simulink library "LibDBC_VCUa_ch1"  (R2024b)
settings: Solver=VariableStepAuto  StartTime=0.0  StopTime=10.0  RelTol=1e-3
undefined symbols (not defined in the file): bit_packing, IO_Blk_Lib_TTC500, IO_CAN_ConfigMsg
libraries: IOBlock_Library_TTC580 x2, simulink x2
(part 1 of 2)
Description:
  | 13-Jun-2024 19:00:134624
settings Model: Creator=Jacob  LastModifiedBy=Jacob

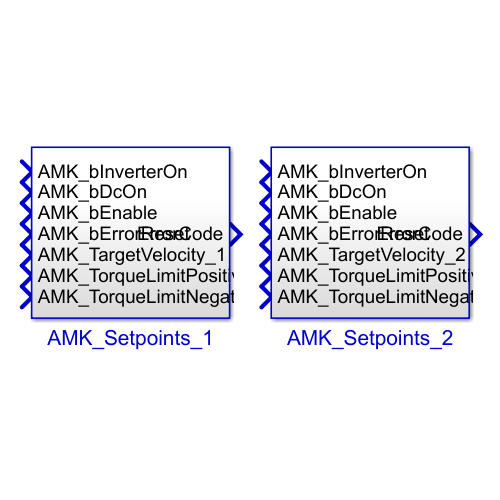
[thumbnail: Simulink's stored preview of the top-level diagram]
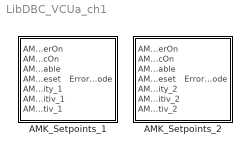
== system LibDBC_VCUa_ch1 ==
  AMK_Setpoints_1 : Subsystem  Priority=0
  AMK_Setpoints_2 : Subsystem  Priority=0

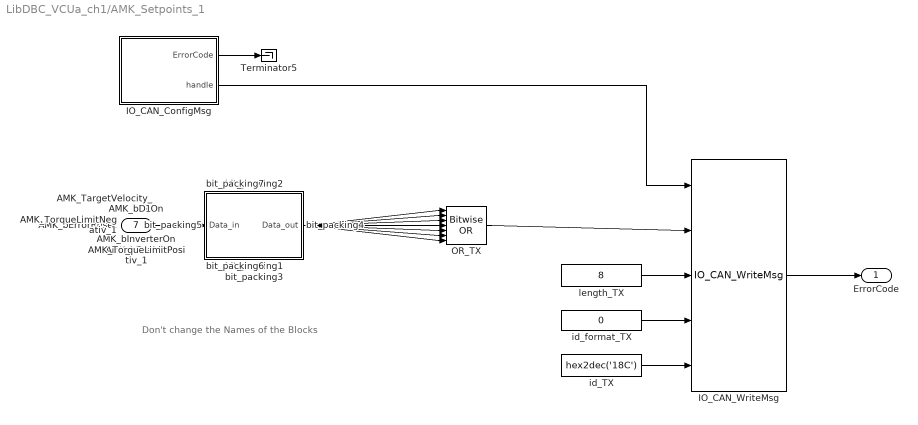
== system LibDBC_VCUa_ch1/AMK_Setpoints_1 ==
  note: Don't change the Names of the Blocks
  AMK_bInverterOn : Inport
  AMK_bDcOn : Inport  Port=2
  AMK_bEnable : Inport  Port=3
  AMK_bErrorReset : Inport  Port=4
  AMK_TargetVelocity_1 : Inport  Port=5
  AMK_TorqueLimitPositiv_1 : Inport  Port=6
  AMK_TorqueLimitNegativ_1 : Inport  Port=7
  IO_CAN_ConfigMsg : Subsystem  mask(IO_CAN_ConfigMsg_Code){SampleTime=-1, ttlib=IO_Blk_Lib_TTC500, ttDescription=IO_CAN_ConfigMsg, tt_iolib_version=0.19, channel=IO_CAN_CHANNEL_1, mode=IO_CAN_MSG_WRITE, id_format=IO_CAN_STD_FRAME, id=0x18C, ac_mask=0x7FF}
      mask help: Configures a message object for the given CAN channel.
      mask init:
      | %
      mask Help: web(which('IO_CAN.h'))
      mask TypeOptions channel: IO_CAN_CHANNEL_0  | IO_CAN_CHANNEL_1 | IO_CAN_CHANNEL_2 | IO_CAN_CHANNEL_3 | IO_CAN_CHANNEL_4 | IO_CAN_CHANNEL_5 | IO_CAN_CHANNEL_6
      mask Callback channel: %
      mask TypeOptions mode: IO_CAN_MSG_READ | IO_CAN_MSG_WRITE
      mask Callback mode: %
      mask TypeOptions id_format: IO_CAN_STD_FRAME | IO_CAN_EXT_FRAME
      mask Callback id_format: %
      mask Callback id: %
      mask Callback ac_mask: %
  IO_CAN_WriteMsg : IOBlock_Library_TTC580/CAN  Blocks TTC580 IOlib/WriteMsg_CAN/IO_CAN_WriteMsg  SampleTime=-1  ttlib=IO_Blk_Lib_TTC500  ttDescription=IO_CAN_WriteMsg  tt_iolib_version=0.19
      settings: SourceProductName=I/O Blocklibrary for TTC580
  OR_TX : simulink/Logic and Bit Operations/Bitwise Operator  logicop=OR  UseBitMask=off  NumInputPorts=7  BitMask=bin2dec('11011001')  BitMaskRealWorld=Stored Integer
  Terminator5 : Terminator
  bit_packing1 : Subsystem  LoadFcn=|  mask(bit_packing_Code){SampleTime=-1, ttlib=IO_Blk_Lib_TTC500, ttDescription=bit_packing, tt_iolib_version=0.26, Endianness=little, Format=unsigned, Inversion=off, Startbit=8, Width_bits=1, Factor=1, Offset=0}
      | try
      | %
      | %Upgrade Information - standard BEGIN
      | new_color = 'blue';
      | new_ver = '0.26';
      | act_ver = get_param(gcb,'tt_iolib_version');
      | if not(strcmp(act_ver,new_ver))
      |     disp(['Upgrade block: ',gcb,char(10),'       Version: ',act_ver,' to ',new_ver]);
      |     %switch - case for specific upgrade information e.g. additional parameter required 
      |     %Change appearance and version information
      |     set_param(gcb,'ForegroundColor',new_color);
      |     set_param(gcb,'tt_iolib_version',new_ver);
      | end
      | %Upgrade Information - standard END
      | catch
      | %Standard catch section BEGIN
      | errordlg('An error occurred in a callback of the TTC580-BlockLib. Please open the Diagnostic Viewer for further details');
      | disp(' ');
      | disp('------------------------------------------------------------');
      | disp('An error occurred in a callback of the TTC580-BlockLib.');
      | disp(['Please check the parameters in the mask of ',gcb]);
      | disp('If you do not encounter any violations, then please '); 
      | disp('copy the following lines and report this to support@ttcontrol.com ');
      | disp('<< begin of error message dump >>');
      | disp(['Version of TTC580-BlockLib: ', get_param(gcb,'tt_iolib_version')]);
      | disp(get_param(gcb,'ttDescription'));
      | disp(gcb);
      | x=lasterror;disp(x.message);
      | disp(get_param(gcb,'MaskValues'));
      | disp(version);
      | disp(computer);
      | disp('<< end of error message dump >>');
      | disp('------------------------------------------------------------');
      | disp(' ');
      | %Standard catch section END
      | end
      mask help:
      | Block to prepare CAN-transmition at specified position within 64bit field.
      | For "Factor" and "Offset" the definition of Vector's CANdb applies:
      | [Physical value] = ( [Raw value] * [Factor] ) + [Offset]
      | with Raw value of a signal being the value as it is transmitted in the CAN-network.
      | Verification capabilities are supported.
      mask init:
      | try
      | %%CT>
      | TAG_loc = get_param(gcb,'Tag');
      | if ~isempty(TAG_loc),[~,y]=regexp(TAG_loc,'(^[a-zA-Z0-9_]*)');
      |     if isempty(y) || y~=builtin('length',(TAG_loc)) %don't use length() alone!
      |         error(['The Tag: ',TAG_loc,' needs to start with a letter and may only contain the characters 0-9,a-Z,_ .']);
      | end,end
      | x=find_system(gcbh,'FollowLinks','on','LookUnderMasks','on','BlockType','S-Function');
      | for i=1:builtin('length',(x)) %don't use length() alone!
      |     set_param(x(i),'Tag',TAG_loc);
      | end
      | %<CT%
      | 
      | catch
      | %Standard catch section BEGIN
      | errordlg('An error occurred in a callback of the TTC580-BlockLib. Please open the Diagnostic Viewer for further details');
      | disp(' ');
      | disp('------------------------------------------------------------');
      | disp('An error occurred in a callback of the TTC580-BlockLib.');
      | disp(['Please check the parameters in the mask of ',gcb]);
      | disp('If you do not encounter any violations, then please '); 
      | disp('copy the following lines and report this to support@ttcontrol.com ');
      | disp('<< begin of error message dump >>');
      | disp(['Version of TTC580-BlockLib: ', get_param(gcb,'tt_iolib_version')]);
      | disp(get_param(gcb,'ttDescription'));
      | disp(gcb);
      | x=lasterror;disp(x.message);
      | disp(get_param(gcb,'MaskValues'));
      | disp(version);
      | disp(computer);
      | disp('<< end of error message dump >>');
      | disp('------------------------------------------------------------');
      | disp(' ');
      | %Standard catch section END
      | end
      mask Help: web([which('usermanual.html'),'#',lower(get_param(gcb,'ttDescription'))])
      mask TypeOptions Endianness: big | little
      mask Callback Endianness: %
      mask TypeOptions Format: unsigned | signed | real32
      mask Callback Format: %
      mask Callback Inversion: %
      mask Callback Startbit: %
      mask Callback Width_bits: %
      mask Callback Factor: %
      mask Callback Offset: %
  bit_packing2 : Subsystem  LoadFcn=|  mask(bit_packing_Code){SampleTime=-1, ttlib=IO_Blk_Lib_TTC500, ttDescription=bit_packing, tt_iolib_version=0.26, Endianness=little, Format=unsigned, Inversion=off, Startbit=9, Width_bits=1, Factor=1, Offset=0}
      | try
      | %
      | %Upgrade Information - standard BEGIN
      | new_color = 'blue';
      | new_ver = '0.26';
      | act_ver = get_param(gcb,'tt_iolib_version');
      | if not(strcmp(act_ver,new_ver))
      |     disp(['Upgrade block: ',gcb,char(10),'       Version: ',act_ver,' to ',new_ver]);
      |     %switch - case for specific upgrade information e.g. additional parameter required 
      |     %Change appearance and version information
      |     set_param(gcb,'ForegroundColor',new_color);
      |     set_param(gcb,'tt_iolib_version',new_ver);
      | end
      | %Upgrade Information - standard END
      | catch
      | %Standard catch section BEGIN
      | errordlg('An error occurred in a callback of the TTC580-BlockLib. Please open the Diagnostic Viewer for further details');
      | disp(' ');
      | disp('------------------------------------------------------------');
      | disp('An error occurred in a callback of the TTC580-BlockLib.');
      | disp(['Please check the parameters in the mask of ',gcb]);
      | disp('If you do not encounter any violations, then please '); 
      | disp('copy the following lines and report this to support@ttcontrol.com ');
      | disp('<< begin of error message dump >>');
      | disp(['Version of TTC580-BlockLib: ', get_param(gcb,'tt_iolib_version')]);
      | disp(get_param(gcb,'ttDescription'));
      | disp(gcb);
      | x=lasterror;disp(x.message);
      | disp(get_param(gcb,'MaskValues'));
      | disp(version);
      | disp(computer);
      | disp('<< end of error message dump >>');
      | disp('------------------------------------------------------------');
      | disp(' ');
      | %Standard catch section END
      | end
      mask help:
      | Block to prepare CAN-transmition at specified position within 64bit field.
      | For "Factor" and "Offset" the definition of Vector's CANdb applies:
      | [Physical value] = ( [Raw value] * [Factor] ) + [Offset]
      | with Raw value of a signal being the value as it is transmitted in the CAN-network.
      | Verification capabilities are supported.
      mask init: same as LibDBC_VCUa_ch1/AMK_Setpoints_1/bit_packing1
      mask Help: web([which('usermanual.html'),'#',lower(get_param(gcb,'ttDescription'))])
      mask TypeOptions Endianness: big | little
      mask Callback Endianness: %
      mask TypeOptions Format: unsigned | signed | real32
      mask Callback Format: %
      mask Callback Inversion: %
      mask Callback Startbit: %
      mask Callback Width_bits: %
      mask Callback Factor: %
      mask Callback Offset: %
  bit_packing3 : Subsystem  LoadFcn=|  mask(bit_packing_Code){SampleTime=-1, ttlib=IO_Blk_Lib_TTC500, ttDescription=bit_packing, tt_iolib_version=0.26, Endianness=little, Format=unsigned, Inversion=off, Startbit=10, Width_bits=1, Factor=1, Offset=0}
      | try
      | %
      | %Upgrade Information - standard BEGIN
      | new_color = 'blue';
      | new_ver = '0.26';
      | act_ver = get_param(gcb,'tt_iolib_version');
      | if not(strcmp(act_ver,new_ver))
      |     disp(['Upgrade block: ',gcb,char(10),'       Version: ',act_ver,' to ',new_ver]);
      |     %switch - case for specific upgrade information e.g. additional parameter required 
      |     %Change appearance and version information
      |     set_param(gcb,'ForegroundColor',new_color);
      |     set_param(gcb,'tt_iolib_version',new_ver);
      | end
      | %Upgrade Information - standard END
      | catch
      | %Standard catch section BEGIN
      | errordlg('An error occurred in a callback of the TTC580-BlockLib. Please open the Diagnostic Viewer for further details');
      | disp(' ');
      | disp('------------------------------------------------------------');
      | disp('An error occurred in a callback of the TTC580-BlockLib.');
      | disp(['Please check the parameters in the mask of ',gcb]);
      | disp('If you do not encounter any violations, then please '); 
      | disp('copy the following lines and report this to support@ttcontrol.com ');
      | disp('<< begin of error message dump >>');
      | disp(['Version of TTC580-BlockLib: ', get_param(gcb,'tt_iolib_version')]);
      | disp(get_param(gcb,'ttDescription'));
      | disp(gcb);
      | x=lasterror;disp(x.message);
      | disp(get_param(gcb,'MaskValues'));
      | disp(version);
      | disp(computer);
      | disp('<< end of error message dump >>');
      | disp('------------------------------------------------------------');
      | disp(' ');
      | %Standard catch section END
      | end
      mask help:
      | Block to prepare CAN-transmition at specified position within 64bit field.
      | For "Factor" and "Offset" the definition of Vector's CANdb applies:
      | [Physical value] = ( [Raw value] * [Factor] ) + [Offset]
      | with Raw value of a signal being the value as it is transmitted in the CAN-network.
      | Verification capabilities are supported.
      mask init: same as LibDBC_VCUa_ch1/AMK_Setpoints_1/bit_packing1
      mask Help: web([which('usermanual.html'),'#',lower(get_param(gcb,'ttDescription'))])
      mask TypeOptions Endianness: big | little
      mask Callback Endianness: %
      mask TypeOptions Format: unsigned | signed | real32
      mask Callback Format: %
      mask Callback Inversion: %
      mask Callback Startbit: %
      mask Callback Width_bits: %
      mask Callback Factor: %
      mask Callback Offset: %
  bit_packing4 : Subsystem  LoadFcn=|  mask(bit_packing_Code){SampleTime=-1, ttlib=IO_Blk_Lib_TTC500, ttDescription=bit_packing, tt_iolib_version=0.26, Endianness=little, Format=unsigned, Inversion=off, Startbit=11, Width_bits=1, Factor=1, Offset=0}
      | try
      | %
      | %Upgrade Information - standard BEGIN
      | new_color = 'blue';
      | new_ver = '0.26';
      | act_ver = get_param(gcb,'tt_iolib_version');
      | if not(strcmp(act_ver,new_ver))
      |     disp(['Upgrade block: ',gcb,char(10),'       Version: ',act_ver,' to ',new_ver]);
      |     %switch - case for specific upgrade information e.g. additional parameter required 
      |     %Change appearance and version information
      |     set_param(gcb,'ForegroundColor',new_color);
      |     set_param(gcb,'tt_iolib_version',new_ver);
      | end
      | %Upgrade Information - standard END
      | catch
      | %Standard catch section BEGIN
      | errordlg('An error occurred in a callback of the TTC580-BlockLib. Please open the Diagnostic Viewer for further details');
      | disp(' ');
      | disp('------------------------------------------------------------');
      | disp('An error occurred in a callback of the TTC580-BlockLib.');
      | disp(['Please check the parameters in the mask of ',gcb]);
      | disp('If you do not encounter any violations, then please '); 
      | disp('copy the following lines and report this to support@ttcontrol.com ');
      | disp('<< begin of error message dump >>');
      | disp(['Version of TTC580-BlockLib: ', get_param(gcb,'tt_iolib_version')]);
      | disp(get_param(gcb,'ttDescription'));
      | disp(gcb);
      | x=lasterror;disp(x.message);
      | disp(get_param(gcb,'MaskValues'));
      | disp(version);
      | disp(computer);
      | disp('<< end of error message dump >>');
      | disp('------------------------------------------------------------');
      | disp(' ');
      | %Standard catch section END
      | end
      mask help:
      | Block to prepare CAN-transmition at specified position within 64bit field.
      | For "Factor" and "Offset" the definition of Vector's CANdb applies:
      | [Physical value] = ( [Raw value] * [Factor] ) + [Offset]
      | with Raw value of a signal being the value as it is transmitted in the CAN-network.
      | Verification capabilities are supported.
      mask init: same as LibDBC_VCUa_ch1/AMK_Setpoints_1/bit_packing1
      mask Help: web([which('usermanual.html'),'#',lower(get_param(gcb,'ttDescription'))])
      mask TypeOptions Endianness: big | little
      mask Callback Endianness: %
      mask TypeOptions Format: unsigned | signed | real32
      mask Callback Format: %
      mask Callback Inversion: %
      mask Callback Startbit: %
      mask Callback Width_bits: %
      mask Callback Factor: %
      mask Callback Offset: %
  bit_packing5 : Subsystem  LoadFcn=|  mask(bit_packing_Code){SampleTime=-1, ttlib=IO_Blk_Lib_TTC500, ttDescription=bit_packing, tt_iolib_version=0.26, Endianness=little, Format=signed, Inversion=off, Startbit=16, Width_bits=16, Factor=1, Offset=0}
      | try
      | %
      | %Upgrade Information - standard BEGIN
      | new_color = 'blue';
      | new_ver = '0.26';
      | act_ver = get_param(gcb,'tt_iolib_version');
      | if not(strcmp(act_ver,new_ver))
      |     disp(['Upgrade block: ',gcb,char(10),'       Version: ',act_ver,' to ',new_ver]);
      |     %switch - case for specific upgrade information e.g. additional parameter required 
      |     %Change appearance and version information
      |     set_param(gcb,'ForegroundColor',new_color);
      |     set_param(gcb,'tt_iolib_version',new_ver);
      | end
      | %Upgrade Information - standard END
      | catch
      | %Standard catch section BEGIN
      | errordlg('An error occurred in a callback of the TTC580-BlockLib. Please open the Diagnostic Viewer for further details');
      | disp(' ');
      | disp('------------------------------------------------------------');
      | disp('An error occurred in a callback of the TTC580-BlockLib.');
      | disp(['Please check the parameters in the mask of ',gcb]);
      | disp('If you do not encounter any violations, then please '); 
      | disp('copy the following lines and report this to support@ttcontrol.com ');
      | disp('<< begin of error message dump >>');
      | disp(['Version of TTC580-BlockLib: ', get_param(gcb,'tt_iolib_version')]);
      | disp(get_param(gcb,'ttDescription'));
      | disp(gcb);
      | x=lasterror;disp(x.message);
      | disp(get_param(gcb,'MaskValues'));
      | disp(version);
      | disp(computer);
      | disp('<< end of error message dump >>');
      | disp('------------------------------------------------------------');
      | disp(' ');
      | %Standard catch section END
      | end
      mask help:
      | Block to prepare CAN-transmition at specified position within 64bit field.
      | For "Factor" and "Offset" the definition of Vector's CANdb applies:
      | [Physical value] = ( [Raw value] * [Factor] ) + [Offset]
      | with Raw value of a signal being the value as it is transmitted in the CAN-network.
      | Verification capabilities are supported.
      mask init: same as LibDBC_VCUa_ch1/AMK_Setpoints_1/bit_packing1
      mask Help: web([which('usermanual.html'),'#',lower(get_param(gcb,'ttDescription'))])
      mask TypeOptions Endianness: big | little
      mask Callback Endianness: %
      mask TypeOptions Format: unsigned | signed | real32
      mask Callback Format: %
      mask Callback Inversion: %
      mask Callback Startbit: %
      mask Callback Width_bits: %
      mask Callback Factor: %
      mask Callback Offset: %
  bit_packing6 : Subsystem  LoadFcn=|  mask(bit_packing_Code){SampleTime=-1, ttlib=IO_Blk_Lib_TTC500, ttDescription=bit_packing, tt_iolib_version=0.26, Endianness=little, Format=signed, Inversion=off, Startbit=32, Width_bits=16, Factor=1, Offset=0}
      | try
      | %
      | %Upgrade Information - standard BEGIN
      | new_color = 'blue';
      | new_ver = '0.26';
      | act_ver = get_param(gcb,'tt_iolib_version');
      | if not(strcmp(act_ver,new_ver))
      |     disp(['Upgrade block: ',gcb,char(10),'       Version: ',act_ver,' to ',new_ver]);
      |     %switch - case for specific upgrade information e.g. additional parameter required 
      |     %Change appearance and version information
      |     set_param(gcb,'ForegroundColor',new_color);
      |     set_param(gcb,'tt_iolib_version',new_ver);
      | end
      | %Upgrade Information - standard END
      | catch
      | %Standard catch section BEGIN
      | errordlg('An error occurred in a callback of the TTC580-BlockLib. Please open the Diagnostic Viewer for further details');
      | disp(' ');
      | disp('------------------------------------------------------------');
      | disp('An error occurred in a callback of the TTC580-BlockLib.');
      | disp(['Please check the parameters in the mask of ',gcb]);
      | disp('If you do not encounter any violations, then please '); 
      | disp('copy the following lines and report this to support@ttcontrol.com ');
      | disp('<< begin of error message dump >>');
      | disp(['Version of TTC580-BlockLib: ', get_param(gcb,'tt_iolib_version')]);
      | disp(get_param(gcb,'ttDescription'));
      | disp(gcb);
      | x=lasterror;disp(x.message);
      | disp(get_param(gcb,'MaskValues'));
      | disp(version);
      | disp(computer);
      | disp('<< end of error message dump >>');
      | disp('------------------------------------------------------------');
      | disp(' ');
      | %Standard catch section END
      | end
      mask help:
      | Block to prepare CAN-transmition at specified position within 64bit field.
      | For "Factor" and "Offset" the definition of Vector's CANdb applies:
      | [Physical value] = ( [Raw value] * [Factor] ) + [Offset]
      | with Raw value of a signal being the value as it is transmitted in the CAN-network.
      | Verification capabilities are supported.
      mask init: same as LibDBC_VCUa_ch1/AMK_Setpoints_1/bit_packing1
      mask Help: web([which('usermanual.html'),'#',lower(get_param(gcb,'ttDescription'))])
      mask TypeOptions Endianness: big | little
      mask Callback Endianness: %
      mask TypeOptions Format: unsigned | signed | real32
      mask Callback Format: %
      mask Callback Inversion: %
      mask Callback Startbit: %
      mask Callback Width_bits: %
      mask Callback Factor: %
      mask Callback Offset: %
  bit_packing7 : Subsystem  LoadFcn=|  mask(bit_packing_Code){SampleTime=-1, ttlib=IO_Blk_Lib_TTC500, ttDescription=bit_packing, tt_iolib_version=0.26, Endianness=little, Format=signed, Inversion=off, Startbit=48, Width_bits=16, Factor=0.01, Offset=0}
      | try
      | %
      | %Upgrade Information - standard BEGIN
      | new_color = 'blue';
      | new_ver = '0.26';
      | act_ver = get_param(gcb,'tt_iolib_version');
      | if not(strcmp(act_ver,new_ver))
      |     disp(['Upgrade block: ',gcb,char(10),'       Version: ',act_ver,' to ',new_ver]);
      |     %switch - case for specific upgrade information e.g. additional parameter required 
      |     %Change appearance and version information
      |     set_param(gcb,'ForegroundColor',new_color);
      |     set_param(gcb,'tt_iolib_version',new_ver);
      | end
      | %Upgrade Information - standard END
      | catch
      | %Standard catch section BEGIN
      | errordlg('An error occurred in a callback of the TTC580-BlockLib. Please open the Diagnostic Viewer for further details');
      | disp(' ');
      | disp('------------------------------------------------------------');
      | disp('An error occurred in a callback of the TTC580-BlockLib.');
      | disp(['Please check the parameters in the mask of ',gcb]);
      | disp('If you do not encounter any violations, then please '); 
      | disp('copy the following lines and report this to support@ttcontrol.com ');
      | disp('<< begin of error message dump >>');
      | disp(['Version of TTC580-BlockLib: ', get_param(gcb,'tt_iolib_version')]);
      | disp(get_param(gcb,'ttDescription'));
      | disp(gcb);
      | x=lasterror;disp(x.message);
      | disp(get_param(gcb,'MaskValues'));
      | disp(version);
      | disp(computer);
      | disp('<< end of error message dump >>');
      | disp('------------------------------------------------------------');
      | disp(' ');
      | %Standard catch section END
      | end
      mask help:
      | Block to prepare CAN-transmition at specified position within 64bit field.
      | For "Factor" and "Offset" the definition of Vector's CANdb applies:
      | [Physical value] = ( [Raw value] * [Factor] ) + [Offset]
      | with Raw value of a signal being the value as it is transmitted in the CAN-network.
      | Verification capabilities are supported.
      mask init: same as LibDBC_VCUa_ch1/AMK_Setpoints_1/bit_packing1
      mask Help: web([which('usermanual.html'),'#',lower(get_param(gcb,'ttDescription'))])
      mask TypeOptions Endianness: big | little
      mask Callback Endianness: %
      mask TypeOptions Format: unsigned | signed | real32
      mask Callback Format: %
      mask Callback Inversion: %
      mask Callback Startbit: %
      mask Callback Width_bits: %
      mask Callback Factor: %
      mask Callback Offset: %
  id_TX : Constant  Value=hex2dec('18C')  OutDataTypeStr=uint32
  id_format_TX : Constant  Value=0  OutDataTypeStr=Inherit: Inherit via back propagation
  length_TX : Constant  Value=8  OutDataTypeStr=Inherit: Inherit via back propagation
  ErrorCode : Outport  VectorParamsAs1DForOutWhenUnconnected=off
  wires:
  id_TX/1 -> IO_CAN_WriteMsg/5
  id_format_TX/1 -> IO_CAN_WriteMsg/4
  length_TX/1 -> IO_CAN_WriteMsg/3
  IO_CAN_ConfigMsg/2(handle) -> IO_CAN_WriteMsg/1
  IO_CAN_ConfigMsg/1(ErrorCode) -> Terminator5/1
  IO_CAN_WriteMsg/1 -> ErrorCode/1
  AMK_bInverterOn/1 -> bit_packing1/1(Data_in)
  bit_packing1/1(Data_out) -> OR_TX/1
  AMK_bDcOn/1 -> bit_packing2/1(Data_in)
  bit_packing2/1(Data_out) -> OR_TX/2
  AMK_bEnable/1 -> bit_packing3/1(Data_in)
  bit_packing3/1(Data_out) -> OR_TX/3
  AMK_bErrorReset/1 -> bit_packing4/1(Data_in)
  bit_packing4/1(Data_out) -> OR_TX/4
  AMK_TargetVelocity_1/1 -> bit_packing5/1(Data_in)
  bit_packing5/1(Data_out) -> OR_TX/5
  AMK_TorqueLimitPositiv_1/1 -> bit_packing6/1(Data_in)
  bit_packing6/1(Data_out) -> OR_TX/6
  AMK_TorqueLimitNegativ_1/1 -> bit_packing7/1(Data_in)
  bit_packing7/1(Data_out) -> OR_TX/7
  OR_TX/1 -> IO_CAN_WriteMsg/2

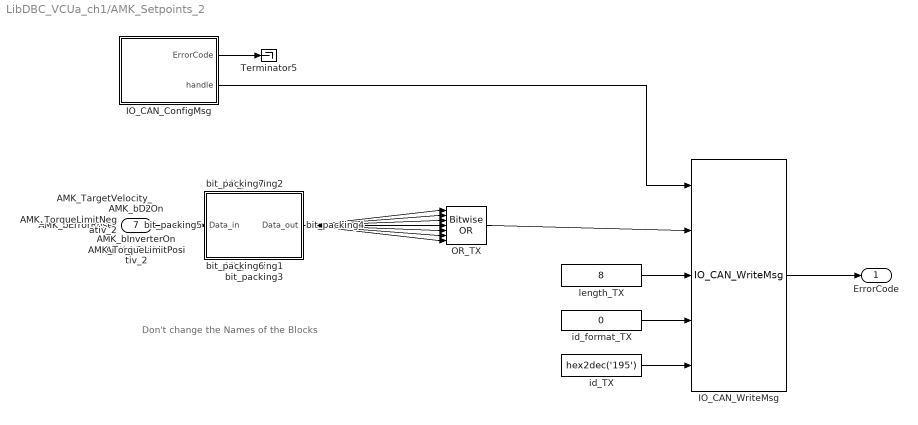
== system LibDBC_VCUa_ch1/AMK_Setpoints_2 ==
  note: Don't change the Names of the Blocks
  AMK_bInverterOn : Inport
  AMK_bDcOn : Inport  Port=2
  AMK_bEnable : Inport  Port=3
  AMK_bErrorReset : Inport  Port=4
  AMK_TargetVelocity_2 : Inport  Port=5
  AMK_TorqueLimitPositiv_2 : Inport  Port=6
  AMK_TorqueLimitNegativ_2 : Inport  Port=7
  IO_CAN_ConfigMsg : Subsystem  mask(IO_CAN_ConfigMsg_Code){SampleTime=-1, ttlib=IO_Blk_Lib_TTC500, ttDescription=IO_CAN_ConfigMsg, tt_iolib_version=0.19, channel=IO_CAN_CHANNEL_1, mode=IO_CAN_MSG_WRITE, id_format=IO_CAN_STD_FRAME, id=0x195, ac_mask=0x7FF}
      mask help: Configures a message object for the given CAN channel.
      mask init:
      | %
      mask Help: web(which('IO_CAN.h'))
      mask TypeOptions channel: IO_CAN_CHANNEL_0  | IO_CAN_CHANNEL_1 | IO_CAN_CHANNEL_2 | IO_CAN_CHANNEL_3 | IO_CAN_CHANNEL_4 | IO_CAN_CHANNEL_5 | IO_CAN_CHANNEL_6
      mask Callback channel: %
      mask TypeOptions mode: IO_CAN_MSG_READ | IO_CAN_MSG_WRITE
      mask Callback mode: %
      mask TypeOptions id_format: IO_CAN_STD_FRAME | IO_CAN_EXT_FRAME
      mask Callback id_format: %
      mask Callback id: %
      mask Callback ac_mask: %
  IO_CAN_WriteMsg : IOBlock_Library_TTC580/CAN  Blocks TTC580 IOlib/WriteMsg_CAN/IO_CAN_WriteMsg  SampleTime=-1  ttlib=IO_Blk_Lib_TTC500  ttDescription=IO_CAN_WriteMsg  tt_iolib_version=0.19
      settings: SourceProductName=I/O Blocklibrary for TTC580
  OR_TX : simulink/Logic and Bit Operations/Bitwise Operator  logicop=OR  UseBitMask=off  NumInputPorts=7  BitMask=bin2dec('11011001')  BitMaskRealWorld=Stored Integer
  Terminator5 : Terminator
  bit_packing1 : Subsystem  LoadFcn=|  mask(bit_packing_Code){SampleTime=-1, ttlib=IO_Blk_Lib_TTC500, ttDescription=bit_packing, tt_iolib_version=0.26, Endianness=little, Format=unsigned, Inversion=off, Startbit=8, Width_bits=1, Factor=1, Offset=0}
      | try
      | %
      | %Upgrade Information - standard BEGIN
      | new_color = 'blue';
      | new_ver = '0.26';
      | act_ver = get_param(gcb,'tt_iolib_version');
      | if not(strcmp(act_ver,new_ver))
      |     disp(['Upgrade block: ',gcb,char(10),'       Version: ',act_ver,' to ',new_ver]);
      |     %switch - case for specific upgrade information e.g. additional parameter required 
      |     %Change appearance and version information
      |     set_param(gcb,'ForegroundColor',new_color);
      |     set_param(gcb,'tt_iolib_version',new_ver);
      | end
      | %Upgrade Information - standard END
      | catch
      | %Standard catch section BEGIN
      | errordlg('An error occurred in a callback of the TTC580-BlockLib. Please open the Diagnostic Viewer for further details');
      | disp(' ');
      | disp('------------------------------------------------------------');
      | disp('An error occurred in a callback of the TTC580-BlockLib.');
      | disp(['Please check the parameters in the mask of ',gcb]);
      | disp('If you do not encounter any violations, then please '); 
      | disp('copy the following lines and report this to support@ttcontrol.com ');
      | disp('<< begin of error message dump >>');
      | disp(['Version of TTC580-BlockLib: ', get_param(gcb,'tt_iolib_version')]);
      | disp(get_param(gcb,'ttDescription'));
      | disp(gcb);
      | x=lasterror;disp(x.message);
      | disp(get_param(gcb,'MaskValues'));
      | disp(version);
      | disp(computer);
      | disp('<< end of error message dump >>');
      | disp('------------------------------------------------------------');
      | disp(' ');
      | %Standard catch section END
      | end
      mask help:
      | Block to prepare CAN-transmition at specified position within 64bit field.
      | For "Factor" and "Offset" the definition of Vector's CANdb applies:
      | [Physical value] = ( [Raw value] * [Factor] ) + [Offset]
      | with Raw value of a signal being the value as it is transmitted in the CAN-network.
      | Verification capabilities are supported.
      mask init: same as LibDBC_VCUa_ch1/AMK_Setpoints_1/bit_packing1
      mask Help: web([which('usermanual.html'),'#',lower(get_param(gcb,'ttDescription'))])
      mask TypeOptions Endianness: big | little
      mask Callback Endianness: %
      mask TypeOptions Format: unsigned | signed | real32
      mask Callback Format: %
      mask Callback Inversion: %
      mask Callback Startbit: %
      mask Callback Width_bits: %
      mask Callback Factor: %
      mask Callback Offset: %
  bit_packing2 : Subsystem  LoadFcn=|  mask(bit_packing_Code){SampleTime=-1, ttlib=IO_Blk_Lib_TTC500, ttDescription=bit_packing, tt_iolib_version=0.26, Endianness=little, Format=unsigned, Inversion=off, Startbit=9, Width_bits=1, Factor=1, Offset=0}
      | try
      | %
      | %Upgrade Information - standard BEGIN
      | new_color = 'blue';
      | new_ver = '0.26';
      | act_ver = get_param(gcb,'tt_iolib_version');
      | if not(strcmp(act_ver,new_ver))
      |     disp(['Upgrade block: ',gcb,char(10),'       Version: ',act_ver,' to ',new_ver]);
      |     %switch - case for specific upgrade information e.g. additional parameter required 
      |     %Change appearance and version information
      |     set_param(gcb,'ForegroundColor',new_color);
      |     set_param(gcb,'tt_iolib_version',new_ver);
      | end
      | %Upgrade Information - standard END
      | catch
      | %Standard catch section BEGIN
      | errordlg('An error occurred in a callback of the TTC580-BlockLib. Please open the Diagnostic Viewer for further details');
      | disp(' ');
      | disp('------------------------------------------------------------');
      | disp('An error occurred in a callback of the TTC580-BlockLib.');
      | disp(['Please check the parameters in the mask of ',gcb]);
      | disp('If you do not encounter any violations, then please '); 
      | disp('copy the following lines and report this to support@ttcontrol.com ');
      | disp('<< begin of error message dump >>');
      | disp(['Version of TTC580-BlockLib: ', get_param(gcb,'tt_iolib_version')]);
      | disp(get_param(gcb,'ttDescription'));
      | disp(gcb);
      | x=lasterror;disp(x.message);
      | disp(get_param(gcb,'MaskValues'));
      | disp(version);
      | disp(computer);
      | disp('<< end of error message dump >>');
      | disp('------------------------------------------------------------');
      | disp(' ');
      | %Standard catch section END
      | end
      mask help:
      | Block to prepare CAN-transmition at specified position within 64bit field.
      | For "Factor" and "Offset" the definition of Vector's CANdb applies:
      | [Physical value] = ( [Raw value] * [Factor] ) + [Offset]
      | with Raw value of a signal being the value as it is transmitted in the CAN-network.
      | Verification capabilities are supported.
      mask init: same as LibDBC_VCUa_ch1/AMK_Setpoints_1/bit_packing1
      mask Help: web([which('usermanual.html'),'#',lower(get_param(gcb,'ttDescription'))])
      mask TypeOptions Endianness: big | little
      mask Callback Endianness: %
      mask TypeOptions Format: unsigned | signed | real32
      mask Callback Format: %
      mask Callback Inversion: %
      mask Callback Startbit: %
      mask Callback Width_bits: %
      mask Callback Factor: %
      mask Callback Offset: %
  bit_packing3 : Subsystem  LoadFcn=|  mask(bit_packing_Code){SampleTime=-1, ttlib=IO_Blk_Lib_TTC500, ttDescription=bit_packing, tt_iolib_version=0.26, Endianness=little, Format=unsigned, Inversion=off, Startbit=10, Width_bits=1, Factor=1, Offset=0}
      | try
      | %
      | %Upgrade Information - standard BEGIN
      | new_color = 'blue';
      | new_ver = '0.26';
      | act_ver = get_param(gcb,'tt_iolib_version');
      | if not(strcmp(act_ver,new_ver))
      |     disp(['Upgrade block: ',gcb,char(10),'       Version: ',act_ver,' to ',new_ver]);
      |     %switch - case for specific upgrade information e.g. additional parameter required 
      |     %Change appearance and version information
      |     set_param(gcb,'ForegroundColor',new_color);
      |     set_param(gcb,'tt_iolib_version',new_ver);
      | end
      | %Upgrade Information - standard END
      | catch
      | %Standard catch section BEGIN
      | errordlg('An error occurred in a callback of the TTC580-BlockLib. Please open the Diagnostic Viewer for further details');
      | disp(' ');
      | disp('------------------------------------------------------------');
      | disp('An error occurred in a callback of the TTC580-BlockLib.');
      | disp(['Please check the parameters in the mask of ',gcb]);
      | disp('If you do not encounter any violations, then please '); 
      | disp('copy the following lines and report this to support@ttcontrol.com ');
      | disp('<< begin of error message dump >>');
      | disp(['Version of TTC580-BlockLib: ', get_param(gcb,'tt_iolib_version')]);
      | disp(get_param(gcb,'ttDescription'));
      | disp(gcb);
      | x=lasterror;disp(x.message);
      | disp(get_param(gcb,'MaskValues'));
      | disp(version);
      | disp(computer);
      | disp('<< end of error message dump >>');
      | disp('------------------------------------------------------------');
      | disp(' ');
      | %Standard catch section END
      | end
      mask help:
      | Block to prepare CAN-transmition at specified position within 64bit field.
      | For "Factor" and "Offset" the definition of Vector's CANdb applies:
      | [Physical value] = ( [Raw value] * [Factor] ) + [Offset]
      | with Raw value of a signal being the value as it is transmitted in the CAN-network.
      | Verification capabilities are supported.
      mask init: same as LibDBC_VCUa_ch1/AMK_Setpoints_1/bit_packing1
      mask Help: web([which('usermanual.html'),'#',lower(get_param(gcb,'ttDescription'))])
      mask TypeOptions Endianness: big | little
      mask Callback Endianness: %
      mask TypeOptions Format: unsigned | signed | real32
      mask Callback Format: %
      mask Callback Inversion: %
      mask Callback Startbit: %
      mask Callback Width_bits: %
      mask Callback Factor: %
      mask Callback Offset: %
  bit_packing4 : Subsystem  LoadFcn=|  mask(bit_packing_Code){SampleTime=-1, ttlib=IO_Blk_Lib_TTC500, ttDescription=bit_packing, tt_iolib_version=0.26, Endianness=little, Format=unsigned, Inversion=off, Startbit=11, Width_bits=1, Factor=1, Offset=0}
      | try
      | %
      | %Upgrade Information - standard BEGIN
      | new_color = 'blue';
      | new_ver = '0.26';
      | act_ver = get_param(gcb,'tt_iolib_version');
      | if not(strcmp(act_ver,new_ver))
      |     disp(['Upgrade block: ',gcb,char(10),'       Version: ',act_ver,' to ',new_ver]);
      |     %switch - case for specific upgrade information e.g. additional parameter required 
      |     %Change appearance and version information
      |     set_param(gcb,'ForegroundColor',new_color);
      |     set_param(gcb,'tt_iolib_version',new_ver);
      | end
      | %Upgrade Information - standard END
      | catch
      | %Standard catch section BEGIN
      | errordlg('An error occurred in a callback of the TTC580-BlockLib. Please open the Diagnostic Viewer for further details');
      | disp(' ');
      | disp('------------------------------------------------------------');
      | disp('An error occurred in a callback of the TTC580-BlockLib.');
      | disp(['Please check the parameters in the mask of ',gcb]);
      | disp('If you do not encounter any violations, then please '); 
      | disp('copy the following lines and report this to support@ttcontrol.com ');
      | disp('<< begin of error message dump >>');
      | disp(['Version of TTC580-BlockLib: ', get_param(gcb,'tt_iolib_version')]);
      | disp(get_param(gcb,'ttDescription'));
      | disp(gcb);
      | x=lasterror;disp(x.message);
      | disp(get_param(gcb,'MaskValues'));
      | disp(version);
      | disp(computer);
      | disp('<< end of error message dump >>');
      | disp('------------------------------------------------------------');
      | disp(' ');
      | %Standard catch section END
      | end
      mask help:
      | Block to prepare CAN-transmition at specified position within 64bit field.
      | For "Factor" and "Offset" the definition of Vector's CANdb applies:
      | [Physical value] = ( [Raw value] * [Factor] ) + [Offset]
      | with Raw value of a signal being the value as it is transmitted in the CAN-network.
      | Verification capabilities are supported.
      mask init: same as LibDBC_VCUa_ch1/AMK_Setpoints_1/bit_packing1
      mask Help: web([which('usermanual.html'),'#',lower(get_param(gcb,'ttDescription'))])
      mask TypeOptions Endianness: big | little
      mask Callback Endianness: %
      mask TypeOptions Format: unsigned | signed | real32
      mask Callback Format: %
      mask Callback Inversion: %
      mask Callback Startbit: %
      mask Callback Width_bits: %
      mask Callback Factor: %
      mask Callback Offset: %
  bit_packing5 : Subsystem  LoadFcn=|  mask(bit_packing_Code){SampleTime=-1, ttlib=IO_Blk_Lib_TTC500, ttDescription=bit_packing, tt_iolib_version=0.26, Endianness=little, Format=signed, Inversion=off, Startbit=16, Width_bits=16, Factor=1, Offset=0}
      | try
      | %
      | %Upgrade Information - standard BEGIN
      | new_color = 'blue';
      | new_ver = '0.26';
      | act_ver = get_param(gcb,'tt_iolib_version');
      | if not(strcmp(act_ver,new_ver))
      |     disp(['Upgrade block: ',gcb,char(10),'       Version: ',act_ver,' to ',new_ver]);
      |     %switch - case for specific upgrade information e.g. additional parameter required 
      |     %Change appearance and version information
      |     set_param(gcb,'ForegroundColor',new_color);
      |     set_param(gcb,'tt_iolib_version',new_ver);
      | end
      | %Upgrade Information - standard END
      | catch
      | %Standard catch section BEGIN
      | errordlg('An error occurred in a callback of the TTC580-BlockLib. Please open the Diagnostic Viewer for further details');
      | disp(' ');
      | disp('------------------------------------------------------------');
      | disp('An error occurred in a callback of the TTC580-BlockLib.');
      | disp(['Please check the parameters in the mask of ',gcb]);
      | disp('If you do not encounter any violations, then please '); 
      | disp('copy the following lines and report this to support@ttcontrol.com ');
      | disp('<< begin of error message dump >>');
      | disp(['Version of TTC580-BlockLib: ', get_param(gcb,'tt_iolib_version')]);
      | disp(get_param(gcb,'ttDescription'));
      | disp(gcb);
      | x=lasterror;disp(x.message);
      | disp(get_param(gcb,'MaskValues'));
      | disp(version);
      | disp(computer);
      | disp('<< end of error message dump >>');
      | disp('------------------------------------------------------------');
      | disp(' ');
      | %Standard catch section END
      | end
      mask help:
      | Block to prepare CAN-transmition at specified position within 64bit field.
      | For "Factor" and "Offset" the definition of Vector's CANdb applies:
      | [Physical value] = ( [Raw value] * [Factor] ) + [Offset]
      | with Raw value of a signal being the value as it is transmitted in the CAN-network.
      | Verification capabilities are supported.
      mask init: same as LibDBC_VCUa_ch1/AMK_Setpoints_1/bit_packing1
      mask Help: web([which('usermanual.html'),'#',lower(get_param(gcb,'ttDescription'))])
      mask TypeOptions Endianness: big | little
      mask Callback Endianness: %
      mask TypeOptions Format: unsigned | signed | real32
      mask Callback Format: %
      mask Callback Inversion: %
      mask Callback Startbit: %
      mask Callback Width_bits: %
      mask Callback Factor: %
      mask Callback Offset: %
  bit_packing6 : Subsystem  LoadFcn=|  mask(bit_packing_Code){SampleTime=-1, ttlib=IO_Blk_Lib_TTC500, ttDescription=bit_packing, tt_iolib_version=0.26, Endianness=little, Format=signed, Inversion=off, Startbit=32, Width_bits=16, Factor=1, Offset=0}
      | try
      | %
      | %Upgrade Information - standard BEGIN
      | new_color = 'blue';
      | new_ver = '0.26';
      | act_ver = get_param(gcb,'tt_iolib_version');
      | if not(strcmp(act_ver,new_ver))
      |     disp(['Upgrade block: ',gcb,char(10),'       Version: ',act_ver,' to ',new_ver]);
      |     %switch - case for specific upgrade information e.g. additional parameter required 
      |     %Change appearance and version information
      |     set_param(gcb,'ForegroundColor',new_color);
      |     set_param(gcb,'tt_iolib_version',new_ver);
      | end
      | %Upgrade Information - standard END
      | catch
      | %Standard catch section BEGIN
      | errordlg('An error occurred in a callback of the TTC580-BlockLib. Please open the Diagnostic Viewer for further details');
      | disp(' ');
      | disp('------------------------------------------------------------');
      | disp('An error occurred in a callback of the TTC580-BlockLib.');
      | disp(['Please check the parameters in the mask of ',gcb]);
      | disp('If you do not encounter any violations, then please '); 
      | disp('copy the following lines and report this to support@ttcontrol.com ');
      | disp('<< begin of error message dump >>');
      | disp(['Version of TTC580-BlockLib: ', get_param(gcb,'tt_iolib_version')]);
      | disp(get_param(gcb,'ttDescription'));
      | disp(gcb);
      | x=lasterror;disp(x.message);
      | disp(get_param(gcb,'MaskValues'));
      | disp(version);
      | disp(computer);
      | disp('<< end of error message dump >>');
      | disp('------------------------------------------------------------');
      | disp(' ');
      | %Standard catch section END
      | end
      mask help:
      | Block to prepare CAN-transmition at specified position within 64bit field.
      | For "Factor" and "Offset" the definition of Vector's CANdb applies:
      | [Physical value] = ( [Raw value] * [Factor] ) + [Offset]
      | with Raw value of a signal being the value as it is transmitted in the CAN-network.
      | Verification capabilities are supported.
      mask init: same as LibDBC_VCUa_ch1/AMK_Setpoints_1/bit_packing1
      mask Help: web([which('usermanual.html'),'#',lower(get_param(gcb,'ttDescription'))])
      mask TypeOptions Endianness: big | little
      mask Callback Endianness: %
      mask TypeOptions Format: unsigned | signed | real32
      mask Callback Format: %
      mask Callback Inversion: %
      mask Callback Startbit: %
      mask Callback Width_bits: %
      mask Callback Factor: %
      mask Callback Offset: %
  bit_packing7 : Subsystem  LoadFcn=|  mask(bit_packing_Code){SampleTime=-1, ttlib=IO_Blk_Lib_TTC500, ttDescription=bit_packing, tt_iolib_version=0.26, Endianness=little, Format=signed, Inversion=off, Startbit=48, Width_bits=16, Factor=0.01, Offset=0}
      | try
      | %
      | %Upgrade Information - standard BEGIN
      | new_color = 'blue';
      | new_ver = '0.26';
      | act_ver = get_param(gcb,'tt_iolib_version');
      | if not(strcmp(act_ver,new_ver))
      |     disp(['Upgrade block: ',gcb,char(10),'       Version: ',act_ver,' to ',new_ver]);
      |     %switch - case for specific upgrade information e.g. additional parameter required 
      |     %Change appearance and version information
      |     set_param(gcb,'ForegroundColor',new_color);
      |     set_param(gcb,'tt_iolib_version',new_ver);
      | end
      | %Upgrade Information - standard END
      | catch
      | %Standard catch section BEGIN
      | errordlg('An error occurred in a callback of the TTC580-BlockLib. Please open the Diagnostic Viewer for further details');
      | disp(' ');
      | disp('------------------------------------------------------------');
      | disp('An error occurred in a callback of the TTC580-BlockLib.');
      | disp(['Please check the parameters in the mask of ',gcb]);
      | disp('If you do not encounter any violations, then please '); 
      | disp('copy the following lines and report this to support@ttcontrol.com ');
      | disp('<< begin of error message dump >>');
      | disp(['Version of TTC580-BlockLib: ', get_param(gcb,'tt_iolib_version')]);
      | disp(get_param(gcb,'ttDescription'));
      | disp(gcb);
      | x=lasterror;disp(x.message);
      | disp(get_param(gcb,'MaskValues'));
      | disp(version);
      | disp(computer);
      | disp('<< end of error message dump >>');
      | disp('------------------------------------------------------------');
      | disp(' ');
      | %Standard catch section END
      | end
      mask help:
      | Block to prepare CAN-transmition at specified position within 64bit field.
      | For "Factor" and "Offset" the definition of Vector's CANdb applies:
      | [Physical value] = ( [Raw value] * [Factor] ) + [Offset]
      | with Raw value of a signal being the value as it is transmitted in the CAN-network.
      | Verification capabilities are supported.
      mask init: same as LibDBC_VCUa_ch1/AMK_Setpoints_1/bit_packing1
      mask Help: web([which('usermanual.html'),'#',lower(get_param(gcb,'ttDescription'))])
      mask TypeOptions Endianness: big | little
      mask Callback Endianness: %
      mask TypeOptions Format: unsigned | signed | real32
      mask Callback Format: %
      mask Callback Inversion: %
      mask Callback Startbit: %
      mask Callback Width_bits: %
      mask Callback Factor: %
      mask Callback Offset: %
  id_TX : Constant  Value=hex2dec('195')  OutDataTypeStr=uint32
  id_format_TX : Constant  Value=0  OutDataTypeStr=Inherit: Inherit via back propagation
  length_TX : Constant  Value=8  OutDataTypeStr=Inherit: Inherit via back propagation
  ErrorCode : Outport  VectorParamsAs1DForOutWhenUnconnected=off
  wires:
  id_TX/1 -> IO_CAN_WriteMsg/5
  id_format_TX/1 -> IO_CAN_WriteMsg/4
  length_TX/1 -> IO_CAN_WriteMsg/3
  IO_CAN_ConfigMsg/2(handle) -> IO_CAN_WriteMsg/1
  IO_CAN_ConfigMsg/1(ErrorCode) -> Terminator5/1
  IO_CAN_WriteMsg/1 -> ErrorCode/1
  AMK_bInverterOn/1 -> bit_packing1/1(Data_in)
  bit_packing1/1(Data_out) -> OR_TX/1
  AMK_bDcOn/1 -> bit_packing2/1(Data_in)
  bit_packing2/1(Data_out) -> OR_TX/2
  AMK_bEnable/1 -> bit_packing3/1(Data_in)
  bit_packing3/1(Data_out) -> OR_TX/3
  AMK_bErrorReset/1 -> bit_packing4/1(Data_in)
  bit_packing4/1(Data_out) -> OR_TX/4
  AMK_TargetVelocity_2/1 -> bit_packing5/1(Data_in)
  bit_packing5/1(Data_out) -> OR_TX/5
  AMK_TorqueLimitPositiv_2/1 -> bit_packing6/1(Data_in)
  bit_packing6/1(Data_out) -> OR_TX/6
  AMK_TorqueLimitNegativ_2/1 -> bit_packing7/1(Data_in)
  bit_packing7/1(Data_out) -> OR_TX/7
  OR_TX/1 -> IO_CAN_WriteMsg/2

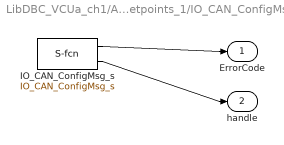
== system LibDBC_VCUa_ch1/AMK_Setpoints_1/IO_CAN_ConfigMsg ==
  IO_CAN_ConfigMsg_s : S-Function  FunctionName=IO_CAN_ConfigMsg_s  Parameters=SampleTime,channel,mode,id_format,id,ac_mask  SFunctionDeploymentMode=off  EnableBusSupport=off
  ErrorCode : Outport  VectorParamsAs1DForOutWhenUnconnected=off
  handle : Outport  Port=2  VectorParamsAs1DForOutWhenUnconnected=off
  wires:
  IO_CAN_ConfigMsg_s/2 -> handle/1
  IO_CAN_ConfigMsg_s/1 -> ErrorCode/1

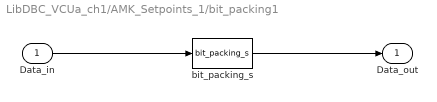
== system LibDBC_VCUa_ch1/AMK_Setpoints_1/bit_packing1 ==
  Data_in : Inport
  bit_packing_s : S-Function  FunctionName=bit_packing_s  Parameters=SampleTime,Endianness,Format,Inversion,Startbit,Width_bits,Factor,Offset  SFunctionDeploymentMode=off  EnableBusSupport=off
  Data_out : Outport  VectorParamsAs1DForOutWhenUnconnected=off
  wires:
  Data_in/1 -> bit_packing_s/1
  bit_packing_s/1 -> Data_out/1

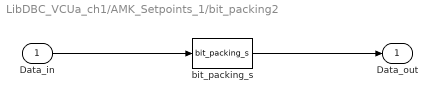
== system LibDBC_VCUa_ch1/AMK_Setpoints_1/bit_packing2 ==
  Data_in : Inport
  bit_packing_s : S-Function  FunctionName=bit_packing_s  Parameters=SampleTime,Endianness,Format,Inversion,Startbit,Width_bits,Factor,Offset  SFunctionDeploymentMode=off  EnableBusSupport=off
  Data_out : Outport  VectorParamsAs1DForOutWhenUnconnected=off
  wires:
  Data_in/1 -> bit_packing_s/1
  bit_packing_s/1 -> Data_out/1

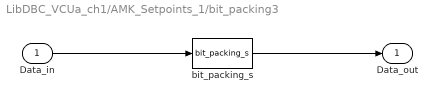
== system LibDBC_VCUa_ch1/AMK_Setpoints_1/bit_packing3 ==
  Data_in : Inport
  bit_packing_s : S-Function  FunctionName=bit_packing_s  Parameters=SampleTime,Endianness,Format,Inversion,Startbit,Width_bits,Factor,Offset  SFunctionDeploymentMode=off  EnableBusSupport=off
  Data_out : Outport  VectorParamsAs1DForOutWhenUnconnected=off
  wires:
  Data_in/1 -> bit_packing_s/1
  bit_packing_s/1 -> Data_out/1

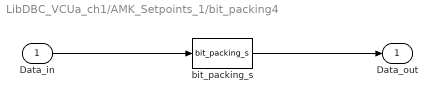
== system LibDBC_VCUa_ch1/AMK_Setpoints_1/bit_packing4 ==
  Data_in : Inport
  bit_packing_s : S-Function  FunctionName=bit_packing_s  Parameters=SampleTime,Endianness,Format,Inversion,Startbit,Width_bits,Factor,Offset  SFunctionDeploymentMode=off  EnableBusSupport=off
  Data_out : Outport  VectorParamsAs1DForOutWhenUnconnected=off
  wires:
  Data_in/1 -> bit_packing_s/1
  bit_packing_s/1 -> Data_out/1

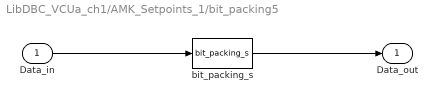
== system LibDBC_VCUa_ch1/AMK_Setpoints_1/bit_packing5 ==
  Data_in : Inport
  bit_packing_s : S-Function  FunctionName=bit_packing_s  Parameters=SampleTime,Endianness,Format,Inversion,Startbit,Width_bits,Factor,Offset  SFunctionDeploymentMode=off  EnableBusSupport=off
  Data_out : Outport  VectorParamsAs1DForOutWhenUnconnected=off
  wires:
  Data_in/1 -> bit_packing_s/1
  bit_packing_s/1 -> Data_out/1

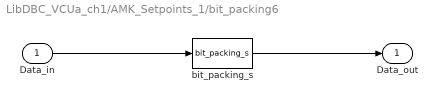
== system LibDBC_VCUa_ch1/AMK_Setpoints_1/bit_packing6 ==
  Data_in : Inport
  bit_packing_s : S-Function  FunctionName=bit_packing_s  Parameters=SampleTime,Endianness,Format,Inversion,Startbit,Width_bits,Factor,Offset  SFunctionDeploymentMode=off  EnableBusSupport=off
  Data_out : Outport  VectorParamsAs1DForOutWhenUnconnected=off
  wires:
  Data_in/1 -> bit_packing_s/1
  bit_packing_s/1 -> Data_out/1
